simulink model "ballbeam_sim"  (R2016b)
settings: Solver=ode45  StartTime=0.0  StopTime=10000  RelTol=1e-3  EnableMultiTasking=on
InitFcn:
  | addpath ./..
  | ballbeam_param
undefined symbols (not defined in the file): ballbeam_animation, P
libraries: simulink x2
settings Model: Creator=beard  LastModifiedBy=beard
settings DataIOCC: LimitDataPoints=on  SaveFormat=Array  SignalLoggingSaveFormat=ModelDataLogs
settings OptimizationCC: ExpressionDepthLimit=2147483647  InitFltsAndDblsToZero=on  LifeSpan=inf
settings DebuggingCC: UnderspecifiedInitializationDetection=Classic  MergeDetectMultiDrivingBlocksExec=none  SolverPrmCheckMsg=warning  FcnCallInpInsideContextMsg=warning  StateNameClashWarn=warning  SFUnexpectedBacktrackingDiag=warning  SFNoUnconditionalDefaultTransitionDiag=warning  SFExecutionAtInitializationDiag=none
settings HardwareCC: ProdBitPerPointer=32  ProdBitPerSizeT=32  ProdBitPerPtrDiffT=32  ProdLargestAtomicFloat=None  ProdIntDivRoundTo=Undefined  ProdEndianess=Unspecified  ProdWordSize=32  ProdHWDeviceType=32-bit Generic
settings ModelReferenceCC: PropagateSignalLabelsOutOfModel=off
settings GRTTargetCC: TargetLangStandard=C89/C90 (ANSI)  GeneratePreprocessorConditionals=Disable all  CombineOutputUpdateFcns=off  GRTInterface=on
settings ConfigComp: CovMetricSettings=dw  CovHtmlReporting=on  CovSaveCumulativeToWorkspaceVar=on  CovSaveSingleToWorkspaceVar=on  CovExternalEMLEnable=off

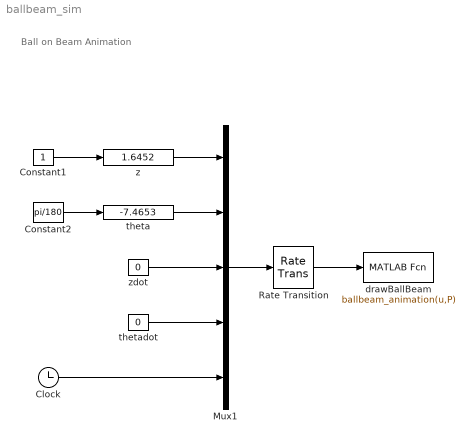
== system ballbeam_sim ==
  note: Ball on Beam Animation
  Clock : Clock
  Constant1 : Constant
  Constant2 : Constant  Value=pi/180
  Mux1 : Mux  Inputs=5
  Rate Transition : RateTransition  OutPortSampleTime=P.t_plot
  drawBallBeam : MATLABFcn  MATLABFcn=ballbeam_animation(u,P)  OutputDimensions=0
  theta : simulink/Math Operations/Slider Gain  low=-180  gain=-7.4653  high=180
  thetadot : Constant  Value=0
  z : simulink/Math Operations/Slider Gain  low=-3  gain=1.6452  high=3
  zdot : Constant  Value=0
  wires:
  Constant1/1 -> z/1
  Constant2/1 -> theta/1
  z/1 -> Mux1/1
  Clock/1 -> Mux1/5
  theta/1 -> Mux1/2
  zdot/1 -> Mux1/3
  thetadot/1 -> Mux1/4
  Mux1/1 -> Rate Transition/1
  Rate Transition/1 -> drawBallBeam/1
